simulink model "Immersion_3"  (Simulink 9.1)
settings: Solver=ode45  StartTime=0.0  StopTime=6  FixedStep=0.01  RelTol=1e-3  EnableMultiTasking=on
model workspace (MAT data in the model file):
  random_seed : num (value not decoded)
undefined symbols (not defined in the file): CafHat, CarHat, K, lam_1, lam_2, Lf, Lr, m, mu, random_seeds, Vel
libraries: simulink x4, Solver_SF x1
settings Model: Creator=xuwei  LastModifiedBy=CK12
settings DataIOCC: LimitDataPoints=on
settings OptimizationCC: ExpressionDepthLimit=2147483647
settings DebuggingCC: SolverPrmCheckMsg=warning  FcnCallInpInsideContextMsg=warning  StateNameClashWarn=warning
settings ConfigComp: CovHtmlReporting=off

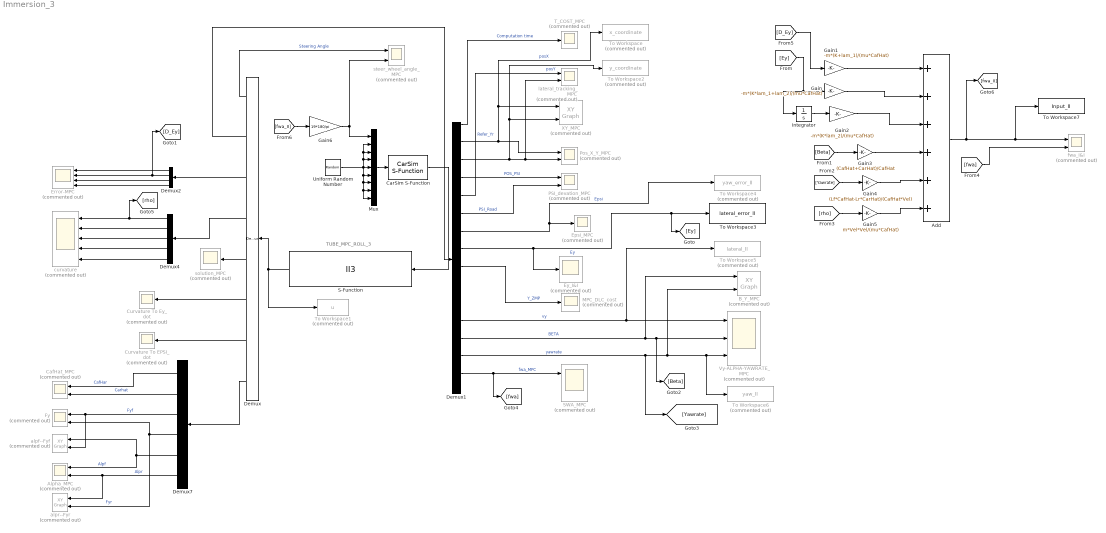
== system Immersion_3 ==
  note: TUBE_MPC_ROLL_3
  Add : Sum  Inputs=++++++
  Alpha_MPC : Scope  Commented=on  NumInputPorts=2
  B_Y_MPC : simulink/Sinks/XY Graph  Commented=on  xmin=-0.1  xmax=0.1  ymin=-0.9  ymax=0.9  st=-1
  CafHat_MPC : Scope  Commented=on  NumInputPorts=2
  CarSim S-Function : Solver_SF/CarSim S-Function  Priority=1  SIMFILE=simfile.sim  Run_RTs=off  vs_state_ind=Run  StopMode_ind=Vehicle Model
  Curvature To EPSI_dot : Scope  Commented=on
  Curvature To Ey_dot : Scope  Commented=on
  Demux : Demux  Outputs=[1 16 4 5 1 5 5 6]
  Demux1 : Demux  Outputs=16
  Demux2 : Demux
  Demux4 : Demux  Outputs=5
  Demux7 : Demux  Outputs=6
  Epsi_MPC : Scope  Commented=on
  Error-MPC : Scope  Commented=on  NumInputPorts=4
  Ey_I&I : Scope  Commented=on
  Fy : Scope  Commented=on  NumInputPorts=2
  Gain : Gain  Gain=-m*(K*lam_1+lam_2)/(mu*CafHat)
  Gain1 : Gain  Gain=-m*(K+lam_1)/(mu*CafHat)
  Gain2 : Gain  Gain=-m*(K*lam_2)/(mu*CafHat)
  Gain3 : Gain  Gain=(CafHat+CarHat)/CafHat
  Gain4 : Gain  Gain=(Lf*CafHat-Lr*CarHat)/(CafHat*Vel)
  Gain5 : Gain  Gain=m*Vel*Vel/(mu*CafHat)
  Gain6 : Gain  Gain=19*180/pi
  Integrator : Integrator
  MPC_DLC_cost : Scope  Commented=on
  Mux : Mux  Inputs=9
  PSI_devation_MPC : Scope  Commented=on  NumInputPorts=2
  Pos_X_Y_MPC : Scope  Commented=on  NumInputPorts=2
  S-Function : S-Function  FunctionName=II3  SFunctionDeploymentMode=off  EnableBusSupport=off
  SWA_MPC : Scope  Commented=on  NumInputPorts=2
  T_COST_MPC : Scope  Commented=on
  To Workspace : ToWorkspace  Commented=on  VariableName=x_coordinate  SampleTime=-1
  To Workspace1 : ToWorkspace  Commented=on  VariableName=u  SaveFormat=Structure  SampleTime=-1
  To Workspace2 : ToWorkspace  Commented=on  VariableName=y_coordinate  SampleTime=-1
  To Workspace3 : ToWorkspace  VariableName=lateral_error_II  SaveFormat=Timeseries  SampleTime=-1
  To Workspace4 : ToWorkspace  Commented=on  VariableName=yaw_error_II  SaveFormat=Timeseries  SampleTime=-1
  To Workspace5 : ToWorkspace  Commented=on  VariableName=lateral_II  SaveFormat=Timeseries  SampleTime=-1
  To Workspace6 : ToWorkspace  Commented=on  VariableName=yaw_II  SaveFormat=Timeseries  SampleTime=-1
  To Workspace7 : ToWorkspace  VariableName=Input_II  SaveFormat=Timeseries  SampleTime=-1
  Uniform Random Number : UniformRandomNumber  Minimum=0.4  Maximum=0.8  Seed=random_seeds  SampleTime=0.1
  Vy-ALPHA-YAWRATE_MPC : Scope  Commented=on  NumInputPorts=3
  XY_MPC : simulink/Sinks/XY Graph  Commented=on  xmin=-10  xmax=180  ymin=-4  ymax=4  st=-1
  alpf--Fyf : simulink/Sinks/XY Graph  Commented=on  xmin=-0.15  xmax=0.15  ymin=-8000  ymax=8000  st=-1
  alpr--Fyr : simulink/Sinks/XY Graph  Commented=on  xmin=-0.1  xmax=0.1  ymin=-6000  ymax=6000  st=-1
  curvature : Scope  Commented=on  NumInputPorts=5
  "fwa_I&I " : Scope  Commented=on  NumInputPorts=2
  lateral_tracking_MPC : Scope  Commented=on  NumInputPorts=2
  "solution_MPC " : Scope  Commented=on
  steer_wheel_angle_MPC : Scope  Commented=on  NumInputPorts=2
  wires:
  CarSim S-Function/1 -> S-Function/1
  S-Function/1 -> Demux/1, To Workspace1/1
  Demux/2 -> Demux1/1
  Demux2/1 -> Error-MPC/1
  Demux2/2 -> [D_Ey], Error-MPC/2
  Demux2/3 -> Error-MPC/3
  Demux2/4 -> Error-MPC/4
  Demux/3 -> Demux2/1
  Demux1/6 -> PSI_devation_MPC/2  "PSI_Road"
  Demux1/14 -> Vy-ALPHA-YAWRATE_MPC/3, To Workspace6/1, B_Y_MPC/2, [Yawrate]  "yawrate"
  Demux1/4 -> PSI_devation_MPC/1  "POS_PSI"
  Demux1/9 -> MPC_DLC_cost/1  "Y_ZMP"
  Demux1/12 -> Vy-ALPHA-YAWRATE_MPC/1, To Workspace5/1  "vy"
  Demux1/13 -> [Beta], Vy-ALPHA-YAWRATE_MPC/2, B_Y_MPC/1  "BETA"
  Demux1/15 -> [fwa], SWA_MPC/1  "fwa_MPC"
  Demux/5 -> "solution_MPC "/1
  Demux4/2 -> curvature/2
  Demux4/3 -> curvature/3
  Demux4/4 -> curvature/4
  Demux4/5 -> curvature/5
  Demux/6 -> Curvature To Ey_dot/1
  Demux/7 -> Curvature To EPSI_dot/1
  Demux/8 -> Demux7/1
  Demux7/1 -> CafHat_MPC/1  "CafHar"
  Demux7/2 -> CafHat_MPC/2  "Carhat"
  Demux7/3 -> Fy/1, alpf--Fyf/2  "Fyf"
  Demux7/4 -> alpr--Fyr/2, Fy/2  "Fyr"
  Demux7/5 -> Alpha_MPC/1, alpf--Fyf/1  "Alpf"
  Demux7/6 -> alpr--Fyr/1, Alpha_MPC/2  "Alpr"
  Demux1/5 -> lateral_tracking_MPC/1  "Refer_Yr"
  Demux1/3 -> Pos_X_Y_MPC/2, lateral_tracking_MPC/2, XY_MPC/2, To Workspace2/1  "posY"
  Demux1/1 -> T_COST_MPC/1  "Computation time"
  Demux1/2 -> Pos_X_Y_MPC/1, XY_MPC/1, To Workspace/1  "posX"
  Demux1/7 -> To Workspace4/1, Epsi_MPC/1  "Epsi"
  Demux/1 -> steer_wheel_angle_MPC/1  "Steering Angle"
  Demux1/8 -> [Ey], To Workspace3/1, Ey_I&I/1  "Ey"
  Demux/4 -> Demux4/1
  Demux4/1 -> [rho], curvature/1
  [D_Ey] -> Gain1/1
  Gain4/1 -> Add/5
  [Ey] -> Integrator/1, Gain/1
  Integrator/1 -> Gain2/1
  [Yawrate] -> Gain4/1
  Add/1 -> [fwa_II], To Workspace7/1, "fwa_I&I "/1
  Gain/1 -> Add/2
  [fwa] -> "fwa_I&I "/2
  Gain3/1 -> Add/4
  Gain1/1 -> Add/1
  [rho] -> Gain5/1
  Gain5/1 -> Add/6
  [Beta] -> Gain3/1
  Gain2/1 -> Add/3
  [fwa_II] -> Gain6/1
  Gain6/1 -> Mux/1, steer_wheel_angle_MPC/2
  Uniform Random Number/1 -> Mux/9, Mux/8, Mux/7, Mux/6, Mux/5, Mux/2, Mux/3, Mux/4
  Mux/1 -> CarSim S-Function/1
